simulink model "Active_Balancing_Subsystem"  (R2020a)
settings: Solver=FixedStepDiscrete  StartTime=0.0  StopTime=10.0  FixedStep=.1  RelTol=1e-3
libraries: simulink x1
settings Model: Creator=Administrator  LastModifiedBy=Administrator
settings OptimizationCC: DefaultParameterBehavior=Inlined  EnhancedBackFolding=on  PassReuseOutputArgsAs=Individual arguments  ZeroExternalMemoryAtStartup=off  ZeroInternalMemoryAtStartup=off  OptimizeBlockOrder=speed  DifferentSizesBufferReuse=on  OptimizationCustomize=off  EfficientTunableParamExpr=on
settings DebuggingCC: ParameterTunabilityLossMsg=error
settings HardwareCC: ProdBitPerPointer=32  ProdBitPerSizeT=32  ProdBitPerPtrDiffT=32  ProdLargestAtomicInteger=Long  ProdLargestAtomicFloat=Double  ProdWordSize=32  ProdHWDeviceType=ARM Compatible->ARM Cortex
settings SFSimCC: MATLABDynamicMemAlloc=off
settings RTWCC: SystemTargetFile=ert.tlc  TemplateMakefile=ert_default_tmf
settings CodeAppCC: ForceParamTrailComments=on  IgnoreCustomStorageClasses=off  OperatorAnnotations=on  SimulinkDataObjDesc=on  SFDataObjDesc=on  InsertBlockDesc=on
settings ERTTargetCC: TargetLangStandard=C99 (ISO)  GenerateSampleERTMain=on  InlinedParameterPlacement=NonHierarchical  ERTCustomFileTemplate=example_file_process.tlc

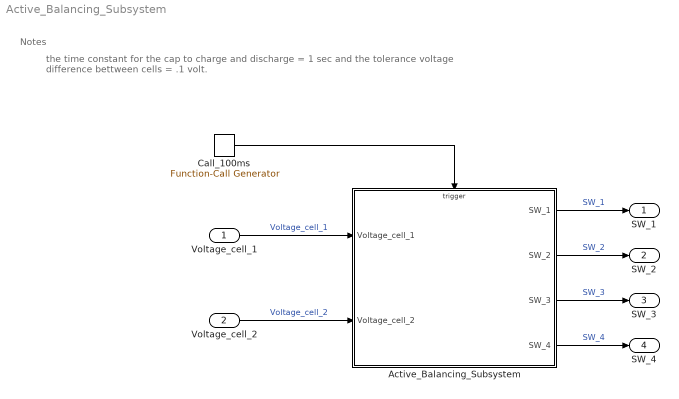
== system Active_Balancing_Subsystem ==
  note: Notes
  note: the time constant for the cap to charge and discharge = 1 sec
      | and the tolerance voltage difference bettween cells = .1 volt.
  Voltage_cell_1 : Inport
  Voltage_cell_2 : Inport  Port=2
  Active_Balancing_Subsystem : Subsystem
  Call_100ms : simulink/Ports & Subsystems/Function-Call Generator  sample_time=1  numberOfIterations=1
  SW_1 : Outport
  SW_2 : Outport  Port=2
  SW_3 : Outport  Port=3
  SW_4 : Outport  Port=4
  wires:
  Active_Balancing_Subsystem/1(SW_1) -> SW_1/1  "SW_1"
  Active_Balancing_Subsystem/2(SW_2) -> SW_2/1  "SW_2"
  Active_Balancing_Subsystem/3(SW_3) -> SW_3/1  "SW_3"
  Active_Balancing_Subsystem/4(SW_4) -> SW_4/1  "SW_4"
  Call_100ms/1 -> Active_Balancing_Subsystem/Trigger
  Voltage_cell_1/1 -> Active_Balancing_Subsystem/1(Voltage_cell_1)  "Voltage_cell_1"
  Voltage_cell_2/1 -> Active_Balancing_Subsystem/2(Voltage_cell_2)  "Voltage_cell_2"

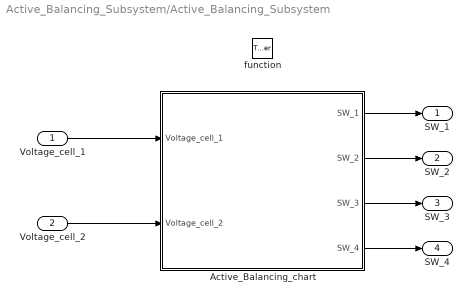
== system Active_Balancing_Subsystem/Active_Balancing_Subsystem ==
  Voltage_cell_1 : Inport
  Voltage_cell_2 : Inport  Port=2
  function : TriggerPort  TriggerType=function-call  VariantControl=Variant
  Active_Balancing_chart : Stateflow chart  TreatAsAtomicUnit=on
  SW_1 : Outport
  SW_2 : Outport  Port=2
  SW_3 : Outport  Port=3
  SW_4 : Outport  Port=4
  wires:
  Active_Balancing_chart/1(SW_1) -> SW_1/1
  Active_Balancing_chart/2(SW_2) -> SW_2/1
  Active_Balancing_chart/3(SW_3) -> SW_3/1
  Voltage_cell_2/1 -> Active_Balancing_chart/2(Voltage_cell_2)
  Voltage_cell_1/1 -> Active_Balancing_chart/1(Voltage_cell_1)
  Active_Balancing_chart/4(SW_4) -> SW_4/1

== stateflow chart Active_Balancing_Subsystem/Active_Balancing_chart ==
  state Need_Balance [function]
    (default) -> (junction 19)
    (junction 19) -> (junction 20) [order 1] : [Voltage_cell_1==Voltage_cell_2]
    (junction 19) -> (junction 21) [order 2] : {Need_Balance_State=1;}
    (junction 20) -> (junction 22) : {Need_Balance_State=0;}
    (junction 22) -> (junction 21)
    (junction 21) -> (junction 23)
  state Decision_Maker
    state SW_Managment
      state Mode_A
        en:
        SW_1=1; SW_3=1;
        du:
        Need_Balance();
        Delta=abs(Voltage_cell_1-Voltage_cell_2);
        ex:
        SW_1=0; SW_3=0;
      state Mode_B
        en:
        SW_2=1; SW_4=1;
        du:
        Need_Balance();
        Delta=abs(Voltage_cell_1-Voltage_cell_2);
        ex:
        SW_2=0; SW_4=0;
      (default) -> Mode_A
      Mode_A -> Mode_B : after(1,sec)
      Mode_B -> Mode_A : after(1,sec)
    state Leader_State
      en,du:
      Delta=abs(Voltage_cell_1-Voltage_cell_2);
      Need_Balance();
      Lowest_Battery();
    (default) -> Leader_State
    Leader_State -> Mode_A [order 1] : [Need_Balance_State==1 && Delta>Target_Delta && lowest==2]
    SW_Managment -> Leader_State : [Voltage_cell_1==Voltage_cell_2]
    Leader_State -> Mode_B [order 2] : [Need_Balance_State==1 && Delta>Target_Delta && lowest==1]
  state Lowest_Battery [function]
    (default) -> (junction 52)
    (junction 52) -> (junction 53) [order 1] : [Voltage_cell_1>Voltage_cell_2]
    (junction 52) -> (junction 54) [order 2]
    (junction 53) -> (junction 58) : {lowest=2;}
    (junction 54) -> (junction 55) [order 1] : [Voltage_cell_2>Voltage_cell_1]
    (junction 54) -> (junction 56) [order 2] : {lowest=0;}
    (junction 55) -> (junction 57) : {lowest=1;}
    (junction 57) -> (junction 56)
    (junction 58) -> (junction 57)
    (junction 56) -> (junction 59)
  (default) -> Decision_Maker
  data: Voltage_cell_1 input single; Voltage_cell_2 input single; SW_1 output boolean; SW_2 output boolean; SW_3 output boolean; SW_4 output boolean; Delta local double; Target_Delta constant double =.1; Need_Balance_State local double; lowest local double
